simulink model "finalcode"  (R2020a)
settings: Solver=FixedStepDiscrete  StartTime=0.0  StopTime=1  FixedStep=0.0005  RelTol=1e-3  EnableMultiTasking=on
undefined symbols (not defined in the file): acc_calmax1, acc_calmax2, acc_calmin1, acc_calmin2, akemancanshu, angle_middle, bre, bre_calmax, bre_calmin, chasuniujvvvv_hou, chasuniujvvvv_qian, chasuuuu, ecucoder_acal, I_AN01_5K1, I_AN03_5V, I_AN04_5V, kd, kddd, ki, kiii, kp, kppp, leftmax, O_SW06_HS1A, P11111, P22222, PIDmodel, PPPP, rightmax, slip, slip_big, slip_little, slipmodel, T_add, T_del, tiaoshi, TTTTTyouren, vvvv, zhiling
libraries: ec5744lib x305, canmsglib x97, simulink x23
(part 7 of 11)

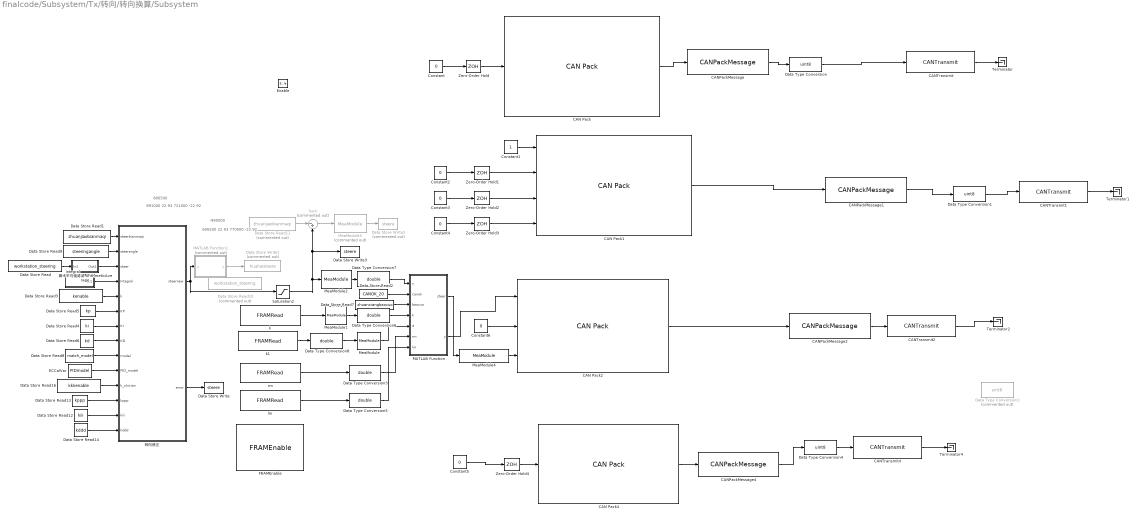
== system finalcode/Subsystem/Tx/转向/转向换算/Subsystem ==
  note: 606500  22.93
      | 770000  -22.92
  note: -990000
  note: 891000  22.93
      | 721000  -22.92
  note: 806500
  Enable : EnablePort
  CAN Pack : canmsglib/CAN Pack  CANdbFile=C:\Users\Liu keliang\Desktop\HRT2023\HRT23赛季刘科良\CANdbc\steering.dbc  MsgList=(none)  MsgName=enable123  MsgIDType=Standard (11-bit identifier)  MsgIdentifier=291  MsgLength=1  Remote=off  ApplyMinMax=off  BusOutput=off  SignalInfo={'enable123','0','8','LE','unsigned','Standard','0','1','0','0','255'}
      settings: SourceProductBaseCode=ME,XP,VN  DataFormat=CANdb specified signals
  CAN Pack1 : canmsglib/CAN Pack  CANdbFile=C:\Users\Liu keliang\Desktop\HRT2023\HRT23赛季刘科良\CANdbc\steering.dbc  MsgList=(none)  MsgName=enable0  MsgIDType=Standard (11-bit identifier)  MsgIdentifier=0  MsgLength=8  Remote=off  ApplyMinMax=off  BusOutput=off  SignalInfo={'enable_00','0','16','LE','unsigned','Standard','0','1','0','0','65535';'enable_00_Copy_1','16','16','LE','unsigned','Standard','0','1','0','0','65535';'enable_00_Copy_2','32','16','LE','unsigned','Standard','0','1','0','0','65535';'enable_00_Copy_3','48','16','LE','unsigned','Standard','0','1','0','0','65535'}
      settings: SourceProductBaseCode=ME,XP,VN  DataFormat=CANdb specified signals
  CAN Pack2 : canmsglib/CAN Pack  CANdbFile=C:\Users\Liu keliang\Desktop\HRT2023\HRT23赛季刘科良\CANdbc\steering.dbc  MsgList=(none)  MsgName=enable401  MsgIDType=Standard (11-bit identifier)  MsgIdentifier=1025  MsgLength=6  Remote=off  ApplyMinMax=off  BusOutput=off  SignalInfo={'enable401','0','8','LE','unsigned','Standard','0','1','0','0','255';'enable401_Copy_1','8','8','LE','unsigned','Standard','0','1','0','0','255';'enable401_Copy_2','16','32','LE','signed','Standard','0','1','0','-2147483648','2147483647'}
      settings: SourceProductBaseCode=ME,XP,VN  DataFormat=CANdb specified signals
  CAN Pack4 : canmsglib/CAN Pack  CANdbFile=C:\Users\Liu keliang\Desktop\HRT2023\HRT23赛季刘科良\CANdbc\steering.dbc  MsgList=(none)  MsgName=enable80  MsgIDType=Standard (11-bit identifier)  MsgIdentifier=128  MsgLength=1  Remote=off  ApplyMinMax=off  BusOutput=off  SignalInfo={'dingshi','0','8','LE','unsigned','Standard','0','1','0','0','255'}
      settings: SourceProductBaseCode=ME,XP,VN  DataFormat=CANdb specified signals
  CANPackMessage : ec5744lib/RapidECU_U4B/04CANCommunication/CANPackMessage  datalength=1  sampletime=-1
      settings: SourceProductName=ECUCoder for MPC5744
  CANPackMessage1 : ec5744lib/RapidECU_U4B/04CANCommunication/CANPackMessage  datalength=8  sampletime=-1
      settings: SourceProductName=ECUCoder for MPC5744
  CANPackMessage2 : ec5744lib/RapidECU_U4B/04CANCommunication/CANPackMessage  datalength=6  sampletime=-1
      settings: SourceProductName=ECUCoder for MPC5744
  CANPackMessage4 : ec5744lib/RapidECU_U4B/04CANCommunication/CANPackMessage  datalength=1  sampletime=-1
      settings: SourceProductName=ECUCoder for MPC5744
  CANTransmit : ec5744lib/RapidECU_U4B/04CANCommunication/CANTransmit  canmodule=2  canbuffer=15  canmessageid=hex2dec('123')  canmessagetype=Standard(11-bit ID)  datalength=1  sampletime=-1
      settings: SourceProductName=ECUCoder for MPC5744
  CANTransmit1 : ec5744lib/RapidECU_U4B/04CANCommunication/CANTransmit  canmodule=2  canbuffer=56  canmessageid=hex2dec('00')  canmessagetype=Standard(11-bit ID)  datalength=8  sampletime=-1
      settings: SourceProductName=ECUCoder for MPC5744
  CANTransmit2 : ec5744lib/RapidECU_U4B/04CANCommunication/CANTransmit  canmodule=2  canbuffer=57  canmessageid=hex2dec('401')  canmessagetype=Standard(11-bit ID)  datalength=6  sampletime=-1
      settings: SourceProductName=ECUCoder for MPC5744
  CANTransmit4 : ec5744lib/RapidECU_U4B/04CANCommunication/CANTransmit  canmodule=2  canbuffer=58  canmessageid=hex2dec('80')  canmessagetype=Standard(11-bit ID)  datalength=1  sampletime=-1
      settings: SourceProductName=ECUCoder for MPC5744
  Constant : Constant  Value=0  SampleTime=-1
  Constant1 : Constant  SampleTime=-1
  Constant{2..4,6} (4 alike) : Constant  Value=0
  Constant5 : Constant  Value=0  SampleTime=-1
  Data Store Read : DataStoreRead  DataStoreName=workstation_steering
  Data Store Read1 : DataStoreRead  DataStoreName=zhuanjiaobianmaqi
  Data Store Read10 : DataStoreRead  Commented=on  DataStoreName=workstation_steering
  Data Store Read11 : DataStoreRead  Commented=on  DataStoreName=zhuanjiaobianmaqi
  Data Store Read12 : DataStoreRead  DataStoreName=kiii
  Data Store Read13 : DataStoreRead  DataStoreName=kppp
  Data Store Read14 : DataStoreRead  DataStoreName=kddd
  Data Store Read16 : DataStoreRead  DataStoreName=kkkenable
  Data Store Read2 : DataStoreRead  DataStoreName=CANOK_20
  Data Store Read3 : DataStoreRead  DataStoreName=kenable
  Data Store Read4 : DataStoreRead  DataStoreName=ki
  Data Store Read5 : DataStoreRead  DataStoreName=kp
  Data Store Read6 : DataStoreRead  DataStoreName=kd
  Data Store Read7 : DataStoreRead  DataStoreName=zhuanxiangbaocuo
  Data Store Read8 : DataStoreRead  DataStoreName=match_model
  Data Store Read9 : DataStoreRead  DataStoreName=steeringangle
  Data Store Write : DataStoreWrite  DataStoreName=steere
  Data Store Write1 : DataStoreWrite  Commented=on  DataStoreName=huahaisteere
  Data Store Write2 : DataStoreWrite  Commented=on  DataStoreName=steere
  Data Store Write3 : DataStoreWrite  DataStoreName=steere
  Data Type Conversion : DataTypeConversion  OutDataTypeStr=uint8
  Data Type Conversion1 : DataTypeConversion  OutDataTypeStr=uint8
  Data Type Conversion2 : DataTypeConversion  Commented=on  OutDataTypeStr=uint8
  Data Type Conversion{3,5..8} (5 alike) : DataTypeConversion  OutDataTypeStr=double
  Data Type Conversion4 : DataTypeConversion  OutDataTypeStr=uint8
  ECCalVar : Constant  InitFcn=ecucoder_acal;  Value=PIDmodel  OutDataTypeStr=Inherit: Inherit via back propagation  SampleTime=-1
  FRAMEnable : ec5744lib/RapidECU_U4B/12EEModule/FRAMEnable  framenable=on
      settings: SourceProductName=ECUCoder for MPC5744
  MATLAB Function : MATLAB Function  TreatAsAtomicUnit=on
  MATLAB Function1 : MATLAB Function  Commented=on  TreatAsAtomicUnit=on
  MeaModule : ec5744lib/RapidECU_U4B/07Calibration/MeaModule  signal=d
      settings: SourceProductName=ECUCoder for MPC5744
  MeaModule1 : ec5744lib/RapidECU_U4B/07Calibration/MeaModule  signal=k
      settings: SourceProductName=ECUCoder for MPC5744
  MeaModule2 : ec5744lib/RapidECU_U4B/07Calibration/MeaModule  signal=steer_toworkstation
      settings: SourceProductName=ECUCoder for MPC5744
  MeaModule3 : ec5744lib/RapidECU_U4B/07Calibration/MeaModule  Commented=on  signal=steer_error
      settings: SourceProductName=ECUCoder for MPC5744
  MeaModule4 : ec5744lib/RapidECU_U4B/07Calibration/MeaModule  signal=zhuanjiaoshuzhi
      settings: SourceProductName=ECUCoder for MPC5744
  Saturation2 : Saturate  UpperLimit=25  LowerLimit=-25
  Sum : Sum  Commented=on  Inputs=|-+
  Terminator{,1..2,4} (4 alike) : Terminator
  Zero-Order Hold{,1..4} (5 alike) : ZeroOrderHold  SampleTime=-1
  integral : Subsystem
  k : ec5744lib/RapidECU_U4B/12EEModule/FRAMRead  buffer=0  sampletime=-1
      settings: SourceProductName=ECUCoder for MPC5744
  k1 : ec5744lib/RapidECU_U4B/12EEModule/FRAMRead  buffer=9  sampletime=-1
      settings: SourceProductName=ECUCoder for MPC5744
  lm : ec5744lib/RapidECU_U4B/12EEModule/FRAMRead  buffer=11  sampletime=-1
      settings: SourceProductName=ECUCoder for MPC5744
  rm : ec5744lib/RapidECU_U4B/12EEModule/FRAMRead  buffer=10  sampletime=-1
      settings: SourceProductName=ECUCoder for MPC5744
  算术平均值滤波 ArithmeticAverage : Subsystem
  转向修正 : MATLAB Function  TreatAsAtomicUnit=on
  wires:
  CANTransmit/1 -> Terminator/1
  Zero-Order Hold2/1 -> CAN Pack1/3
  MATLAB Function/2(y) -> CAN Pack2/1
  CAN Pack1/1 -> CANPackMessage1/1
  CANTransmit2/1 -> Terminator2/1
  CANPackMessage4/1 -> Data Type Conversion4/1
  CAN Pack2/1 -> CANPackMessage2/1
  CANTransmit1/1 -> Terminator1/1
  Constant/1 -> Zero-Order Hold/1
  Data Type Conversion1/1 -> CANTransmit1/1
  Constant6/1 -> CAN Pack2/2
  CANTransmit4/1 -> Terminator4/1
  Data Type Conversion/1 -> CANTransmit/1
  Zero-Order Hold/1 -> CAN Pack/1
  CANPackMessage/1 -> Data Type Conversion/1
  Data Type Conversion4/1 -> CANTransmit4/1
  Constant4/1 -> Zero-Order Hold3/1
  CAN Pack/1 -> CANPackMessage/1
  CANPackMessage1/1 -> Data Type Conversion1/1
  Constant5/1 -> Zero-Order Hold4/1
  CAN Pack4/1 -> CANPackMessage4/1
  Constant3/1 -> Zero-Order Hold2/1
  Constant2/1 -> Zero-Order Hold1/1
  Constant1/1 -> CAN Pack1/1
  Zero-Order Hold4/1 -> CAN Pack4/1
  Zero-Order Hold1/1 -> CAN Pack1/2
  CANPackMessage2/1 -> CANTransmit2/1
  Zero-Order Hold3/1 -> CAN Pack1/4
  MATLAB Function/1(steer) -> MeaModule4/1
  Data Store Read/1 -> 算术平均值滤波 ArithmeticAverage/1(In1)
  Data Store Read1/1 -> 转向修正/1(steerbianmaqi)
  转向修正/2(error) -> Data Store Write/1
  Data Store Read2/1 -> MATLAB Function/2(canok)
  Data Store Read5/1 -> 转向修正/6(KP)
  Data Store Read4/1 -> 转向修正/7(KI)
  Data Store Read3/1 -> 转向修正/5(k)
  Data Store Read6/1 -> 转向修正/8(KD)
  MATLAB Function1/1(y) -> Data Store Write1/1
  Data Store Read7/1 -> MATLAB Function/3(baocuo)
  Data Store Read8/1 -> 转向修正/9(model)
  Data Store Read9/1 -> 转向修正/2(steerangle)
  rm/1 -> Data Type Conversion3/1
  lm/1 -> Data Type Conversion5/1
  MeaModule/1 -> MATLAB Function/5(d)
  k/1 -> MeaModule1/1
  MeaModule1/1 -> Data Type Conversion6/1
  转向修正/1(steernew) -> MATLAB Function1/1(u), Saturation2/1
  MeaModule2/1 -> Data Type Conversion7/1
  Data Store Read11/1 -> Sum/1
  Sum/1 -> MeaModule3/1
  MeaModule3/1 -> Data Store Write2/1
  Data Type Conversion3/1 -> MATLAB Function/6(rm)
  Data Type Conversion5/1 -> MATLAB Function/7(lm)
  Data Type Conversion6/1 -> MATLAB Function/4(k)
  MeaModule4/1 -> CAN Pack2/3
  Data Type Conversion7/1 -> MATLAB Function/1(x)
  ECCalVar/1 -> 转向修正/10(PID_model)
  integral/1(Out1) -> 转向修正/4(Integral)
  算术平均值滤波 ArithmeticAverage/1(Out1) -> 转向修正/3(steer)
  k1/1 -> Data Type Conversion8/1
  Data Type Conversion8/1 -> MeaModule/1
  Data Store Read16/1 -> 转向修正/11(k_zhixian)
  Data Store Read13/1 -> 转向修正/12(kppp)
  Data Store Read12/1 -> 转向修正/13(kiii)
  Data Store Read14/1 -> 转向修正/14(kddd)
  Saturation2/1 -> Sum/2, Data Store Write3/1, MeaModule2/1

== system finalcode/Subsystem/Tx/转向/转向换算/Subsystem1 ==
  y1 : Inport
  y2 : Inport  Port=2
  Enable : EnablePort
  CAN Pack5 : canmsglib/CAN Pack  CANdbFile=C:\Users\Liu keliang\Desktop\HRT2023\HRT23赛季刘科良\CANdbc\zhuanxiangresetting.dbc  MsgList=(none)  MsgName=reseting  MsgIDType=Standard (11-bit identifier)  MsgIdentifier=1537  MsgLength=8  Remote=off  ApplyMinMax=off  BusOutput=off  SignalInfo={'reseting1','0','32','LE','unsigned','Standard','0','1','0','-Inf','Inf';'reseting2','32','32','LE','unsigned','Standard','0','1','0','-Inf','Inf'}
      settings: SourceProductBaseCode=ME,XP,VN  DataFormat=CANdb specified signals
  CANPackMessage3 : ec5744lib/RapidECU_U4B/04CANCommunication/CANPackMessage  datalength=8  sampletime=-1
      settings: SourceProductName=ECUCoder for MPC5744
  CANTransmit3 : ec5744lib/RapidECU_U4B/04CANCommunication/CANTransmit  canmodule=2  canbuffer=60  canmessageid=hex2dec('601')  canmessagetype=Standard(11-bit ID)  datalength=8  sampletime=-1
      settings: SourceProductName=ECUCoder for MPC5744
  Data Type Conversion3 : DataTypeConversion  OutDataTypeStr=uint8
  Terminator3 : Terminator
  wires:
  CAN Pack5/1 -> CANPackMessage3/1
  y1/1 -> CAN Pack5/1
  CANTransmit3/1 -> Terminator3/1
  Data Type Conversion3/1 -> CANTransmit3/1
  CANPackMessage3/1 -> Data Type Conversion3/1
  y2/1 -> CAN Pack5/2

== system finalcode/Subsystem/run/analog_input/无人意图转译/无人 ==
  Data Store Write : DataStoreWrite  DataStoreName=escmax
  Max : MinMax  Function=max  Inputs=4
  Subsystem1 : Subsystem
  右前油压 : DataStoreWrite  DataStoreName=oral_pressure_rightfront
  右后油压 : DataStoreWrite  DataStoreName=oral_pressure_rightbehind
  左前油压 : DataStoreWrite  DataStoreName=oral_pressure_leftfront
  左后油压 : DataStoreWrite  DataStoreName=oral_pressure_leftbehind
  期望加速度 : DataStoreWrite  Commented=on  DataStoreName=acc_expired
  期望纵向加速度 : Outport
  wires:
  Subsystem1/1(期望纵向加速度) -> 期望纵向加速度/1, 期望加速度/1
  Subsystem1/2(输出左前制动力) -> Max/1, 左前油压/1
  Subsystem1/4(输出左后制动力) -> Max/3, 左后油压/1
  Subsystem1/3(输出右前制动力) -> Max/2, 右前油压/1
  Subsystem1/5(输出右后制动力) -> Max/4, 右后油压/1
  Max/1 -> Data Store Write/1

== system finalcode/Subsystem/run/analog_input/有人/Subsystem1 ==
  note: 标定
  acc_signal : Inport
  Constant : Constant  Value=0
  Data Store Read : DataStoreRead  DataStoreName=V_Kalman
  Data Type Conversion : DataTypeConversion  OutMin=[0]  OutMax=[1]  OutDataTypeStr=double
  Divide1 : Product  Inputs=**  OutDataTypeStr=uint16
  ECCalVar : Constant  InitFcn=ecucoder_acal;  Value=T_add  OutDataTypeStr=Inherit: Inherit via back propagation  SampleTime=-1
  ECCalVar1 : Constant  InitFcn=ecucoder_acal;  Value=T_del  OutDataTypeStr=Inherit: Inherit via back propagation  SampleTime=-1
  ECCalVar2 : Constant  InitFcn=ecucoder_acal;  Value=zhiling  OutDataTypeStr=Inherit: Inherit via back propagation  SampleTime=-1
  MATLAB Function : MATLAB Function  TreatAsAtomicUnit=on
  MATLAB Function1 : MATLAB Function  TreatAsAtomicUnit=on
  Saturation3 : Saturate  UpperLimit=2100  LowerLimit=0
  Saturation4 : Saturate  UpperLimit=1  LowerLimit=0
  Sum : Sum  Inputs=|++-
  Sum1 : Sum  Inputs=+--
  normal : MATLAB Function  Commented=on  TreatAsAtomicUnit=on
  TP : Outport
  wires:
  Data Type Conversion/1 -> Saturation4/1
  acc_signal/1 -> Data Type Conversion/1
  Saturation4/1 -> Divide1/2
  Sum/1 -> Divide1/1
  ECCalVar1/1 -> Sum/3
  ECCalVar/1 -> Sum/1
  Saturation3/1 -> Sum/2
  Data Store Read/1 -> MATLAB Function/1(v)
  MATLAB Function/1(T) -> Saturation3/1
  Divide1/1 -> Sum1/1
  Constant/1 -> Sum1/2
  Sum1/1 -> MATLAB Function1/1(T)
  MATLAB Function1/1(TP) -> TP/1
  ECCalVar2/1 -> Sum1/3

== system finalcode/Subsystem/run/analog_input/有人/功率限制 ==
  M_zuoqian : Inport
  M_youqian : Inport  Port=2
  M_zuohou : Inport  Port=3
  M_youhou : Inport  Port=4
  Data Store Read4 : DataStoreRead  DataStoreName=dianji_velcoity_zuoqian
  Data Store Read5 : DataStoreRead  DataStoreName=dianji_velcoity_youhou
  Data Store Read6 : DataStoreRead  DataStoreName=dianji_velcoity_youqian
  Data Store Read7 : DataStoreRead  DataStoreName=dianji_velcoity_zuohou
  Data Store Write : DataStoreWrite  DataStoreName=Tzuoqian
  Data Store Write1 : DataStoreWrite  DataStoreName=Tyouqian
  Data Store Write2 : DataStoreWrite  DataStoreName=Tzuohou
  Data Store Write3 : DataStoreWrite  DataStoreName=Tyouhou
  MATLAB Function : MATLAB Function  TreatAsAtomicUnit=on
  Product{,1..7} (8 alike) : Product
  wires:
  M_youqian/1 -> Product5/1, Product1/1
  M_zuohou/1 -> Product6/1, Product2/1
  M_youhou/1 -> Product7/1, Product3/1
  Data Store Read4/1 -> Product/2
  Data Store Read7/1 -> Product2/2
  Data Store Read5/1 -> Product3/2
  Data Store Read6/1 -> Product1/2
  Product/1 -> MATLAB Function/1(u1)
  Product1/1 -> MATLAB Function/2(u2)
  Product2/1 -> MATLAB Function/3(u3)
  Product3/1 -> MATLAB Function/4(u4)
  MATLAB Function/1(y) -> Product7/2, Product6/2, Product5/2, Product4/2
  M_zuoqian/1 -> Product4/1, Product/1
  Product4/1 -> Data Store Write/1
  Product5/1 -> Data Store Write1/1
  Product6/1 -> Data Store Write2/1
  Product7/1 -> Data Store Write3/1

== system finalcode/Subsystem/run/analog_input/有人/功率限制jiandan ==
  M_zuoqian : Inport
  M_youqian : Inport  Port=2
  M_zuohou : Inport  Port=3
  M_youhou : Inport  Port=4
  Data Store Read4 : DataStoreRead  DataStoreName=dianji_velcoity_zuoqian
  Data Store Read5 : DataStoreRead  DataStoreName=dianji_velcoity_youhou
  Data Store Read6 : DataStoreRead  DataStoreName=dianji_velcoity_youqian
  Data Store Read7 : DataStoreRead  DataStoreName=dianji_velcoity_zuohou
  Data Store Write : DataStoreWrite  DataStoreName=Tzuoqian
  Data Store Write1 : DataStoreWrite  DataStoreName=Tyouqian
  Data Store Write2 : DataStoreWrite  DataStoreName=Tzuohou
  Data Store Write3 : DataStoreWrite  DataStoreName=Tyouhou
  MATLAB Function : MATLAB Function  TreatAsAtomicUnit=on
  Product{,1..7} (8 alike) : Product
  Saturation{1..4} (4 alike) : Saturate  UpperLimit=2100  LowerLimit=0
  wires:
  M_youqian/1 -> Product5/1, Product1/1
  M_zuohou/1 -> Product6/1, Product2/1
  M_youhou/1 -> Product7/1, Product3/1
  Data Store Read4/1 -> Product/2
  Data Store Read7/1 -> Product2/2
  Data Store Read5/1 -> Product3/2
  Data Store Read6/1 -> Product1/2
  Product/1 -> MATLAB Function/1(u1)
  Product1/1 -> MATLAB Function/2(u2)
  Product2/1 -> MATLAB Function/3(u3)
  Product3/1 -> MATLAB Function/4(u4)
  MATLAB Function/1(y) -> Product7/2, Product6/2, Product5/2, Product4/2
  M_zuoqian/1 -> Product4/1, Product/1
  Product4/1 -> Saturation3/1
  Saturation3/1 -> Data Store Write/1
  Product5/1 -> Saturation1/1
  Saturation1/1 -> Data Store Write1/1
  Product6/1 -> Saturation2/1
  Saturation2/1 -> Data Store Write2/1
  Product7/1 -> Saturation4/1
  Saturation4/1 -> Data Store Write3/1

== system finalcode/Subsystem/run/analog_input/有人/扭矩分配 ==
  note: 前后扭矩分配k
  fengzhiniuju : Inport
  Constant2 : Constant  Value=10
  Data Store Read7 : DataStoreRead  DataStoreName=acc_calibration
  Enabled Subsystem : Subsystem  TreatAsAtomicUnit=on
  MATLAB Function : MATLAB Function  TreatAsAtomicUnit=on
  MATLAB Function3 : MATLAB Function  TreatAsAtomicUnit=on
  Saturation : Saturate  UpperLimit=2100  LowerLimit=0
  Saturation1 : Saturate  UpperLimit=2100  LowerLimit=0
  zuoqian : Outport
  youqian : Outport  Port=2
  zuohou : Outport  Port=3
  youhou : Outport  Port=4
  wires:
  MATLAB Function/1(M_qian) -> Saturation1/1
  fengzhiniuju/1 -> MATLAB Function/1(M)
  MATLAB Function/2(M_hou) -> Saturation/1
  Constant2/1 -> MATLAB Function/3(k)
  MATLAB Function3/1(youhou) -> youhou/1
  MATLAB Function3/2(youqian) -> youqian/1
  MATLAB Function3/3(zuohou) -> zuohou/1
  MATLAB Function3/4(zuoqian) -> zuoqian/1
  Data Store Read7/1 -> MATLAB Function/2(ax)
  Enabled Subsystem/1(y) -> MATLAB Function3/3(M)
  Saturation1/1 -> MATLAB Function3/1(M_qian)
  Saturation/1 -> MATLAB Function3/2(M_hou)

== system finalcode/Subsystem/run/analog_input/有人/扭矩分配jiandan ==
  note: 后面加入载荷转移，向心差扭
  note: 前后扭矩分配k
  fengzhiniuju : Inport
  Constant2 : Constant
  Constant3 : Constant
  Data Store Read2 : DataStoreRead  Commented=on  DataStoreName=shucai_ax
  Data Store Read3 : DataStoreRead  Commented=on  DataStoreName=shucai_ay
  MATLAB Function1 : MATLAB Function  Commented=on  TreatAsAtomicUnit=on
  MATLAB Function3 : MATLAB Function  TreatAsAtomicUnit=on
  M_back : Constant  Value=1.3
  M_front : Constant  Value=0.7
  Product1 : Product
  Product2 : Product
  k : Constant  Value=0
  zuoqian : Outport
  youqian : Outport  Port=2
  zuohou : Outport  Port=3
  youhou : Outport  Port=4
  wires:
  MATLAB Function3/1(youhou) -> youhou/1
  MATLAB Function3/2(youqian) -> youqian/1
  MATLAB Function3/3(zuohou) -> zuohou/1
  MATLAB Function3/4(zuoqian) -> zuoqian/1
  k/1 -> MATLAB Function3/3(M)
  Product1/1 -> MATLAB Function3/1(M_qian)
  Product2/1 -> MATLAB Function3/2(M_hou)
  M_front/1 -> Product1/2
  Constant2/1 -> MATLAB Function3/5(zuo)
  Constant3/1 -> MATLAB Function3/4(you)
  fengzhiniuju/1 -> Product2/2, MATLAB Function1/1(fengzhiniuju), Product1/1
  M_back/1 -> Product2/1
  Data Store Read2/1 -> MATLAB Function1/2(ax)
  Data Store Read3/1 -> MATLAB Function1/3(ay)

== system finalcode/Subsystem/run/analog_input/有人/踏板标定 ==
  AnalogInput : ec5744lib/RapidECU_U4B/01BasicInput/AnalogInput  channel=52:I_AN03_5V  sampletime=-1
      settings: SourceProductName=ECUCoder for MPC5744
  AnalogInput1 : ec5744lib/RapidECU_U4B/01BasicInput/AnalogInput  channel=53:I_AN04_5V  sampletime=-1
      settings: SourceProductName=ECUCoder for MPC5744
  AnalogInput2 : ec5744lib/RapidECU_U4B/01BasicInput/AnalogInput  Commented=on  channel=34:I_AN01_5K1  sampletime=-1
      settings: SourceProductName=ECUCoder for MPC5744
  Data Store Write1 : DataStoreWrite  DataStoreName=acc_calibration
  Data Store Write2 : DataStoreWrite  DataStoreName=bre_calibration
  ECCalVar1 : Constant  InitFcn=ecucoder_acal;  Value=acc_calmax1  OutDataTypeStr=double  SampleTime=-1
  ECCalVar2 : Constant  InitFcn=ecucoder_acal;  Value=acc_calmin1  OutDataTypeStr=double  SampleTime=-1
  ECCalVar3 : Constant  InitFcn=ecucoder_acal;  Value=acc_calmax2  OutDataTypeStr=double  SampleTime=-1
  ECCalVar4 : Constant  InitFcn=ecucoder_acal;  Value=acc_calmin2  OutDataTypeStr=double  SampleTime=-1
  ECCalVar5 : Constant  Commented=on  InitFcn=ecucoder_acal;  Value=bre_calmax  OutDataTypeStr=double  SampleTime=-1
  ECCalVar6 : Constant  Commented=on  InitFcn=ecucoder_acal;  Value=bre_calmin  OutDataTypeStr=double  SampleTime=-1
  ECCalVar7 : Constant  InitFcn=ecucoder_acal;  Value=bre  OutDataTypeStr=double  SampleTime=-1
  FRAMEnable : ec5744lib/RapidECU_U4B/12EEModule/FRAMEnable  Commented=on  framenable=off
      settings: SourceProductName=ECUCoder for MPC5744
  MATLAB Function : MATLAB Function  TreatAsAtomicUnit=on
  MATLAB Function1 : MATLAB Function  Commented=on  TreatAsAtomicUnit=on
  MATLAB Function2 : MATLAB Function  TreatAsAtomicUnit=on
  MeaModule1 : ec5744lib/RapidECU_U4B/07Calibration/MeaModule  signal=acc_ori_line1
      settings: SourceProductName=ECUCoder for MPC5744
  MeaModule2 : ec5744lib/RapidECU_U4B/07Calibration/MeaModule  signal=acc_ori_line2
      settings: SourceProductName=ECUCoder for MPC5744
  MeaModule3 : ec5744lib/RapidECU_U4B/07Calibration/MeaModule  signal=guiyi
      settings: SourceProductName=ECUCoder for MPC5744
  MeaModule5 : ec5744lib/RapidECU_U4B/07Calibration/MeaModule  Commented=on  signal=bre_ori_sig
      settings: SourceProductName=ECUCoder for MPC5744
  MeaModule6 : ec5744lib/RapidECU_U4B/07Calibration/MeaModule  signal=acc_result2
      settings: SourceProductName=ECUCoder for MPC5744
  MeaModule8 : ec5744lib/RapidECU_U4B/07Calibration/MeaModule  signal=acc_result1
      settings: SourceProductName=ECUCoder for MPC5744
  MeaModule9 : ec5744lib/RapidECU_U4B/07Calibration/MeaModule  signal=bre_result
      settings: SourceProductName=ECUCoder for MPC5744
  Saturation4 : Saturate  UpperLimit=1  LowerLimit=0
  Subsystem : Subsystem  Commented=on
  Subsystem1 : Subsystem  Commented=on
  无人制动标志位 : DataStoreRead  DataStoreName=wurenzhidongdeng
  算术平均值滤波 ArithmeticAverage1 : Subsystem
  踏板冲突 : MATLAB Function  TreatAsAtomicUnit=on
  踏板冲突1 : MATLAB Function  Commented=on  TreatAsAtomicUnit=on
  acc : Outport
  bre : Outport  Port=2
  wires:
  AnalogInput/1 -> MeaModule1/1
  AnalogInput2/1 -> MeaModule5/1
  MeaModule5/1 -> MATLAB Function1/1(u)
  AnalogInput1/1 -> MeaModule2/1
  MeaModule1/1 -> MATLAB Function/1(u)
  MeaModule2/1 -> MATLAB Function2/1(u)
  MeaModule9/1 -> bre/1, Data Store Write2/1, 踏板冲突/3(bre_ori_sig)
  ECCalVar3/1 -> MATLAB Function2/3(max)
  MATLAB Function2/1(y) -> MeaModule6/1
  ECCalVar1/1 -> MATLAB Function/3(max)
  ECCalVar4/1 -> MATLAB Function2/2(min)
  MATLAB Function/1(y) -> MeaModule8/1
  ECCalVar2/1 -> MATLAB Function/2(min)
  Subsystem1/1(y) -> Subsystem/Enable
  MeaModule6/1 -> 踏板冲突/2(acc_fin_sig2)
  ECCalVar6/1 -> MATLAB Function1/2(min)
  ECCalVar5/1 -> MATLAB Function1/3(max)
  踏板冲突/1(y) -> Saturation4/1
  MeaModule3/1 -> acc/1
  ECCalVar7/1 -> 踏板冲突/4(bre)
  无人制动标志位/1 -> MeaModule9/1
  Saturation4/1 -> Data Store Write1/1, 算术平均值滤波 ArithmeticAverage1/1(In1)
  MeaModule8/1 -> 踏板冲突/1(acc_fin_sig1)
  算术平均值滤波 ArithmeticAverage1/1(angle) -> MeaModule3/1

== system finalcode/Subsystem/run/analog_input/有人/限滑 ==
  note: 左转是正
  zuoqian : Inport
  youqian : Inport  Port=2
  zuohou : Inport  Port=3
  youhou : Inport  Port=4
  Data Store Read : DataStoreRead  DataStoreName=shucai_ax
  Enabled Subsystem : Subsystem  TreatAsAtomicUnit=on
  Enabled Subsystem1 : Subsystem  TreatAsAtomicUnit=on
  MATLAB Function : MATLAB Function  TreatAsAtomicUnit=on
  Switch{,1..3} (4 alike) : Switch  Criteria=u2 > Threshold  Threshold=0.5
  M_zuoqian : Outport
  M_youqian : Outport  Port=2
  M_zuohou : Outport  Port=3
  M_youhou : Outport  Port=4
  wires:
  zuoqian/1 -> Enabled Subsystem1/1(zuoqian), Enabled Subsystem/1(zuoqian)
  zuohou/1 -> Enabled Subsystem1/3(zuohou), Enabled Subsystem/3(zuohou)
  youhou/1 -> Enabled Subsystem1/4(youhou), Enabled Subsystem/4(youhou)
  youqian/1 -> Enabled Subsystem1/2(youqian), Enabled Subsystem/2(youqian)
  Data Store Read/1 -> MATLAB Function/1(u)
  MATLAB Function/1(y) -> Switch2/2, Switch3/2, Switch1/2, Switch/2
  Enabled Subsystem/1(M_zuoqian) -> Switch/1
  Enabled Subsystem1/1(M_zuoqian) -> Switch/3
  Enabled Subsystem/4(M_youhou) -> Switch3/1
  Enabled Subsystem1/4(M_youhou) -> Switch3/3
  Enabled Subsystem1/3(M_zuohou) -> Switch2/3
  Enabled Subsystem/3(M_zuohou) -> Switch2/1
  Enabled Subsystem/2(M_youqian) -> Switch1/1
  Enabled Subsystem1/2(M_youqian) -> Switch1/3
  Switch/1 -> M_zuoqian/1
  Switch3/1 -> M_youhou/1
  Switch1/1 -> M_youqian/1
  Switch2/1 -> M_zuohou/1

== system finalcode/Subsystem/run/ctrl/Subsystem1/control_strategy ==
  TP : Inport
  Data Store Read1 : DataStoreRead  DataStoreName=workstation_steering
  Data Store Read2 : DataStoreRead  DataStoreName=slipyouhou
  Data Store Read4 : DataStoreRead  DataStoreName=workstation_steering
  Data Store Read5 : DataStoreRead  DataStoreName=slipzuohou
  Data Store Read6 : DataStoreRead  DataStoreName=slipyuoqian
  Data Store Read7 : DataStoreRead  DataStoreName=slipzuoqian
  E,H : MATLAB Function  Commented=on  TreatAsAtomicUnit=on
  MATLAB Function : MATLAB Function  Commented=on  TreatAsAtomicUnit=on
  MATLAB Function1 : MATLAB Function  TreatAsAtomicUnit=on
  MATLAB Function2 : MATLAB Function  Commented=on  TreatAsAtomicUnit=on
  MATLAB Function3 : MATLAB Function  TreatAsAtomicUnit=on
  MPC : MATLAB Function  Commented=on  TreatAsAtomicUnit=on
  Subsystem : Subsystem  Commented=on
  Switch{,1..3} (4 alike) : Switch  Criteria=u2 > Threshold
  差速 : Subsystem
  滑模控制 : MATLAB Function  TreatAsAtomicUnit=on
  限滑 : Subsystem
  youhou : Outport
  youqian : Outport  Port=2
  zuohou : Outport  Port=3
  zuoqian : Outport  Port=4
  wires:
  TP/1 -> 差速/1(u), 限滑/1(In1)
  Data Store Read4/1 -> MATLAB Function1/1(angle)
  MATLAB Function1/1(y) -> Switch2/2, Switch3/2, Switch1/2, Switch/2
  限滑/1(youhou) -> Switch/3
  限滑/2(youqian) -> Switch1/3
  限滑/3(zuohou) -> Switch2/3
  限滑/4(zuoqian) -> Switch3/3
  MATLAB Function2/1(A) -> E,H/1(A)
  MATLAB Function2/2(B) -> E,H/2(B)
  MATLAB Function2/3(Q) -> E,H/3(Q)
  MATLAB Function2/4(R) -> E,H/4(R)
  MATLAB Function2/5(F) -> E,H/5(F)
  MATLAB Function2/6(N) -> E,H/6(N)
  差速/1(youhou) -> Switch/1
  差速/2(youqian) -> Switch1/1
  差速/3(zuohou) -> Switch2/1
  差速/4(zuoqian) -> Switch3/1
  Data Store Read1/1 -> MATLAB Function3/1(angle)
  MATLAB Function3/1(y) -> 差速/Enable
  Data Store Read7/1 -> 滑模控制/1(slip_ratio_fl)
  Switch/1 -> 滑模控制/8(driver_torque_cmd_rr)
  Data Store Read2/1 -> 滑模控制/4(slip_ratio_rr)
  Data Store Read6/1 -> 滑模控制/2(slip_ratio_fr)
  Switch3/1 -> 滑模控制/5(driver_torque_cmd_fl)
  Data Store Read5/1 -> 滑模控制/3(slip_ratio_rl)
  Switch1/1 -> 滑模控制/6(driver_torque_cmd_fr)
  Switch2/1 -> 滑模控制/7(driver_torque_cmd_rl)
  滑模控制/4(torque_cmd_rr) -> youhou/1
  滑模控制/2(torque_cmd_fr) -> youqian/1
  滑模控制/3(torque_cmd_rl) -> zuohou/1
  滑模控制/1(torque_cmd_fl) -> zuoqian/1

== system finalcode/Subsystem/Rx/工作站/Subsystem1/Subsystem1/Subsystem ==
  ID : Inport
  msg : Inport  Port=2
  CAN Unpack : canmsglib/CAN Unpack  CANdbFile=C:\Users\Liu keliang\Desktop\HRT2023\HRT23赛季刘科良\CANdbc\INSWORKSTATION.dbc  MsgList=(none)  MsgName=ins  MsgIDType=Standard (11-bit identifier)  MsgIdentifier=33  MsgLength=8  SignalInfo={'Vx','32','16','LE','unsigned','Standard','0','1','0','0','65535';'Vy','48','16','LE','unsigned','Standard','0','1','0','0','65535';'ax','0','8','LE','signed','Standard','0','1','0','-128','127';'ay','8','16','LE','signed','Standard','0','1','0','-32768','32767';'az','24','8','LE','signed','Standard','0','1','0','-128','127'}  IDPort=off  TimestampPort=off  ErrorPort=off  RemotePort=off  LengthPort=off  StatusPort=off  ApplyMinMax=off
      settings: SourceProductBaseCode=ME,XP,VN  DataFormat=CANdb specified signals
  CANUnPackMessage : ec5744lib/RapidECU_U4B/04CANCommunication/CANUnPackMessage  datalength=8  canmessagetype=Standard(11-bit ID)  sampletime=-1
      settings: SourceProductName=ECUCoder for MPC5744
  Data Store Write1 : DataStoreWrite  DataStoreName=ACC_X
  Data Store Write2 : DataStoreWrite  DataStoreName=ACC_Y
  Data Store Write3 : DataStoreWrite  DataStoreName=ACC_Z
  Data Store Write4 : DataStoreWrite  DataStoreName=V_Y
  Data Store Write5 : DataStoreWrite  DataStoreName=V_X
  wires:
  msg/1 -> CANUnPackMessage/2
  CANUnPackMessage/1 -> CAN Unpack/1
  ID/1 -> CANUnPackMessage/1
  CAN Unpack/2 -> Data Store Write4/1
  CAN Unpack/1 -> Data Store Write5/1
  CAN Unpack/3 -> Data Store Write1/1
  CAN Unpack/5 -> Data Store Write3/1
  CAN Unpack/4 -> Data Store Write2/1

== system finalcode/Subsystem/Rx/工作站/Subsystem3/Subsystem/Subsystem ==
  Data Store Read : DataStoreRead  DataStoreName=CANOK_20
  Delay : Delay  DelayLength=1
  Delay1 : Delay
  Delay10 : Delay  DelayLength=11
  Delay11 : Delay  DelayLength=12
  Delay12 : Delay  DelayLength=13
  Delay13 : Delay  DelayLength=14
  Delay14 : Delay  DelayLength=15
  Delay15 : Delay  DelayLength=16
  Delay16 : Delay  DelayLength=17
  Delay17 : Delay  DelayLength=25
  Delay18 : Delay  DelayLength=18
  Delay19 : Delay  DelayLength=19
  Delay2 : Delay  DelayLength=3
  Delay20 : Delay  DelayLength=20
  Delay21 : Delay  DelayLength=21
  Delay22 : Delay  DelayLength=22
  Delay23 : Delay  DelayLength=26
  Delay24 : Delay  DelayLength=24
  Delay25 : Delay  DelayLength=27
  Delay3 : Delay  DelayLength=4
  Delay4 : Delay  DelayLength=5
  Delay5 : Delay  DelayLength=6
  Delay6 : Delay  DelayLength=7
  Delay7 : Delay  DelayLength=8
  Delay8 : Delay  DelayLength=9
  Delay9 : Delay  DelayLength=10
  OR : Logic  Operator=OR  Inputs=27  IconShape=distinctive  AllPortsSameDT=off  OutDataTypeStr=boolean
  Out1 : Outport
  wires:
  Delay2/1 -> OR/2
  Delay/1 -> OR/4
  Data Store Read/1 -> Delay23/1, Delay25/1, Delay17/1, Delay24/1, Delay22/1, Delay21/1, Delay20/1, Delay19/1, Delay18/1, Delay16/1, Delay15/1, Delay14/1, Delay13/1, Delay12/1, Delay11/1, Delay10/1, Delay8/1, Delay6/1, Delay5/1, Delay7/1, Delay9/1, OR/5, Delay3/1, Delay2/1, Delay1/1, Delay/1, Delay4/1
  Delay5/1 -> OR/7
  Delay1/1 -> OR/3
  Delay9/1 -> OR/11
  Delay7/1 -> OR/9
  Delay3/1 -> OR/1
  Delay8/1 -> OR/8
  Delay6/1 -> OR/6
  Delay4/1 -> OR/10
  OR/1 -> Out1/1
  Delay10/1 -> OR/12
  Delay11/1 -> OR/13
  Delay12/1 -> OR/14
  Delay13/1 -> OR/15
  Delay14/1 -> OR/16
  Delay15/1 -> OR/17
  Delay16/1 -> OR/18
  Delay18/1 -> OR/19
  Delay19/1 -> OR/20
  Delay20/1 -> OR/21
  Delay21/1 -> OR/22
  Delay22/1 -> OR/23
  Delay24/1 -> OR/24
  Delay17/1 -> OR/25
  Delay23/1 -> OR/27
  Delay25/1 -> OR/26

== system finalcode/Subsystem/Tx/TX控制器/扭矩/TEST/Subsystem ==
  Enable : EnablePort
  CAN Pack1 : canmsglib/CAN Pack  CANdbFile=C:\Users\Liu keliang\Desktop\HRT2023\HRT23赛季刘科良\CANdbc\TEST.dbc  MsgList=(none)  MsgName=TEST  MsgIDType=Standard (11-bit identifier)  MsgIdentifier=153  MsgLength=5  Remote=off  ApplyMinMax=off  BusOutput=off  SignalInfo={'M','16','8','LE','signed','Standard','0','1','0','-Inf','Inf';'X2D','32','8','LE','signed','Standard','0','1','0','-Inf','Inf';'a','0','8','LE','signed','Standard','0','1','0','-Inf','Inf';'deltv','8','8','LE','signed','Standard','0','1','0','-Inf','Inf';'niuju','24','8','LE','signed','Standard','0','1','0','-Inf','Inf'}
      settings: SourceProductBaseCode=ME,XP,VN  DataFormat=CANdb specified signals
  CANPackMessage1 : ec5744lib/RapidECU_U4B/04CANCommunication/CANPackMessage  datalength=5  sampletime=-1
      settings: SourceProductName=ECUCoder for MPC5744
  CANTransmit : ec5744lib/RapidECU_U4B/04CANCommunication/CANTransmit  canmodule=0  canbuffer=63  canmessageid=hex2dec('99')  canmessagetype=Standard(11-bit ID)  datalength=5  sampletime=-1
      settings: SourceProductName=ECUCoder for MPC5744
  Data Store Read : DataStoreRead  DataStoreName=a
  Data Store Read1 : DataStoreRead  DataStoreName=ve
  Data Store Read2 : DataStoreRead  DataStoreName=M
  Data Store Read3 : DataStoreRead  DataStoreName=acc
  Data Store Read4 : DataStoreRead  DataStoreName=dianji_velcoity_zuoqian
  Data Type Conversion1 : DataTypeConversion  OutDataTypeStr=uint8
  Terminator : Terminator
  wires:
  Data Store Read4/1 -> CAN Pack1/1
  CANTransmit/1 -> Terminator/1
  Data Store Read3/1 -> CAN Pack1/3
  CANPackMessage1/1 -> Data Type Conversion1/1
  Data Store Read2/1 -> CAN Pack1/5
  Data Type Conversion1/1 -> CANTransmit/1
  Data Store Read1/1 -> CAN Pack1/4
  Data Store Read/1 -> CAN Pack1/2
  CAN Pack1/1 -> CANPackMessage1/1

== system finalcode/Subsystem/Tx/TX控制器/控制器发送/184左前1/算术平均值滤波 ArithmeticAverage5 ==
  In1 : Inport
  Constant : Constant  Value=10
  Divide : Product  Inputs=*/
  Sum of Elements : Sum  Inputs=+
  Tapped Delay : simulink/Discrete/Tapped Delay  vinit=0.0  samptime=-1  NumDelays=10  DelayOrder=Oldest  includeCurrent=off
  angle : Outport
  wires:
  Tapped Delay/1 -> Sum of Elements/1
  In1/1 -> Tapped Delay/1
  Divide/1 -> angle/1
  Sum of Elements/1 -> Divide/1
  Constant/1 -> Divide/2

== system finalcode/Subsystem/Tx/TX控制器/控制器发送/184左前1/能量回收功率限制 ==
  note: Tniujv
  note: U
  note: Iq
  Constant1 : Constant  Value=2
  Constant24 : Constant  Value=1000
  Data Store Read1 : DataStoreRead  DataStoreName=er_T_lf
  Data Store Read2 : DataStoreRead  DataStoreName=match_model
  Data Store Read23 : DataStoreRead  DataStoreName=match_model
  Data Store Read25 : DataStoreRead  DataStoreName=er_v_lf
  Data Store Read3 : DataStoreRead  DataStoreName=oral_pressure_leftfront
  Data Store Read4 : DataStoreRead  DataStoreName=Power_recovery
  Data Store Read5 : DataStoreRead  DataStoreName=Negativ_T
  Data Store Read6 : DataStoreRead  DataStoreName=Power_recovery_xunji
  Data Store Read7 : DataStoreRead  DataStoreName=Power_recovery_zhixian
  Data Store Read8 : DataStoreRead  DataStoreName=workstation_status
  Divide : Product  Inputs=*/
  Divide1 : Product  Inputs=***/
  Divide2 : Product  Inputs=**
  Gain : Gain  Gain=100
  Gain1 : Gain  Gain=1.5
  MATLAB Function : MATLAB Function  TreatAsAtomicUnit=on
  MATLAB Function1 : MATLAB Function  TreatAsAtomicUnit=on
  MeaModule : ec5744lib/RapidECU_U4B/07Calibration/MeaModule  signal=NT3
      settings: SourceProductName=ECUCoder for MPC5744
  P功率 : MATLAB Function  TreatAsAtomicUnit=on
  Saturation : Saturate  UpperLimit=0  LowerLimit=-1500
  Saturation1 : Saturate  UpperLimit=1500  LowerLimit=-1500
  Saturation2 : Saturate  UpperLimit=0  LowerLimit=-1500
  Sqrt : Sqrt  SaturateOnIntegerOverflow=on
  扭矩常量Kr  N/A : Constant  Value=0.26
  油压传感器 : DataStoreRead  DataStoreName=ebszhidongyouya
  电压常数Ke V/kU/min : Constant  Value=18.8
  T : Outport
  wires:
  Data Store Read25/1 -> Divide1/1
  电压常数Ke V/kU/min/1 -> Divide1/2
  Constant24/1 -> Divide1/4
  Sqrt/1 -> Divide1/3
  Constant1/1 -> Sqrt/1
  油压传感器/1 -> MATLAB Function/1(youya)
  Divide1/1 -> Divide/2
  Divide/1 -> Divide2/1, MATLAB Function1/3(L_Iq)
  扭矩常量Kr  N/A/1 -> Divide2/2
  MATLAB Function/1(T) -> Gain1/1
  Data Store Read1/1 -> MATLAB Function1/2(Iq)
  Divide2/1 -> Gain/1
  Gain/1 -> Saturation1/1
  MATLAB Function1/1(T) -> Saturation2/1
  Data Store Read2/1 -> MATLAB Function/2(model)
  Data Store Read8/1 -> MATLAB Function/3(status)
  Data Store Read3/1 -> MATLAB Function/4(wurenyouya)
  Data Store Read5/1 -> MATLAB Function/5(Negativ_T)
  Saturation/1 -> MeaModule/1
  Gain1/1 -> Saturation/1
  Saturation1/1 -> MATLAB Function1/4(L_er_T)
  Saturation2/1 -> T/1
  P功率/1(y) -> Divide/1
  Data Store Read23/1 -> P功率/4(model)
  Data Store Read4/1 -> P功率/1(P)
  Data Store Read6/1 -> P功率/2(P1)
  MeaModule/1 -> MATLAB Function1/1(er_T)
  Data Store Read7/1 -> P功率/3(P2)

== system finalcode/Subsystem/Tx/TX控制器/控制器发送/185右前1/算术平均值滤波 ArithmeticAverage5 ==
  In1 : Inport
  Constant : Constant  Value=10
  Divide : Product  Inputs=*/
  Sum of Elements : Sum  Inputs=+
  Tapped Delay : simulink/Discrete/Tapped Delay  vinit=0.0  samptime=-1  NumDelays=10  DelayOrder=Oldest  includeCurrent=off
  angle : Outport
  wires:
  Tapped Delay/1 -> Sum of Elements/1
  In1/1 -> Tapped Delay/1
  Divide/1 -> angle/1
  Sum of Elements/1 -> Divide/1
  Constant/1 -> Divide/2

== system finalcode/Subsystem/Tx/TX控制器/控制器发送/185右前1/能量回收功率限制 ==
  note: U
  note: Iq
  Constant1 : Constant  Value=2
  Constant24 : Constant  Value=1000
  Data Store Read1 : DataStoreRead  DataStoreName=er_T_rf
  Data Store Read2 : DataStoreRead  DataStoreName=match_model
  Data Store Read23 : DataStoreRead  DataStoreName=match_model
  Data Store Read25 : DataStoreRead  DataStoreName=er_v_rf
  Data Store Read3 : DataStoreRead  DataStoreName=oral_pressure_rightfront
  Data Store Read4 : DataStoreRead  DataStoreName=Power_recovery
  Data Store Read5 : DataStoreRead  DataStoreName=Negativ_T
  Data Store Read6 : DataStoreRead  DataStoreName=Power_recovery_xunji
  Data Store Read7 : DataStoreRead  DataStoreName=Power_recovery_zhixian
  Data Store Read8 : DataStoreRead  DataStoreName=workstation_status
  Divide : Product  Inputs=*/
  Divide1 : Product  Inputs=***/
  Divide2 : Product  Inputs=**
  Gain : Gain  Gain=100
  Gain1 : Gain  Gain=1.5
  MATLAB Function : MATLAB Function  TreatAsAtomicUnit=on
  MATLAB Function1 : MATLAB Function  TreatAsAtomicUnit=on
  MATLAB Function2 : MATLAB Function  TreatAsAtomicUnit=on
  Saturation : Saturate  UpperLimit=0  LowerLimit=-1500
  Saturation1 : Saturate  UpperLimit=1500  LowerLimit=-1500
  Saturation2 : Saturate  UpperLimit=0  LowerLimit=-1500
  Sqrt : Sqrt  SaturateOnIntegerOverflow=on
  扭矩常量Kr  N/A : Constant  Value=0.26
  油压传感器 : DataStoreRead  DataStoreName=ebszhidongyouya
  电压常数Ke V/kU/min : Constant  Value=18.8
  T : Outport
  wires:
  Data Store Read25/1 -> Divide1/1
  电压常数Ke V/kU/min/1 -> Divide1/2
  Constant24/1 -> Divide1/4
  Sqrt/1 -> Divide1/3
  Constant1/1 -> Sqrt/1
  Divide1/1 -> Divide/2
  Divide/1 -> MATLAB Function1/3(L_Iq), Divide2/1
  扭矩常量Kr  N/A/1 -> Divide2/2
  MATLAB Function/1(T) -> Gain1/1
  Data Store Read1/1 -> MATLAB Function1/2(Iq)
  Divide2/1 -> Gain/1
  Gain/1 -> Saturation1/1
  MATLAB Function1/1(T) -> Saturation2/1
  油压传感器/1 -> MATLAB Function/1(youya)
  Data Store Read3/1 -> MATLAB Function/4(wurenyouya)
  Data Store Read8/1 -> MATLAB Function/3(status)
  Data Store Read2/1 -> MATLAB Function/2(model)
  Data Store Read5/1 -> MATLAB Function/5(Negativ_T)
  Saturation/1 -> MATLAB Function1/1(er_T)
  Gain1/1 -> Saturation/1
  Saturation1/1 -> MATLAB Function1/4(L_er_T)
  Saturation2/1 -> T/1
  MATLAB Function2/1(y) -> Divide/1
  Data Store Read23/1 -> MATLAB Function2/4(model)
  Data Store Read4/1 -> MATLAB Function2/1(P)
  Data Store Read6/1 -> MATLAB Function2/2(P1)
  Data Store Read7/1 -> MATLAB Function2/3(P2)

== system finalcode/Subsystem/Tx/TX控制器/控制器发送/188右后1/算术平均值滤波 ArithmeticAverage5 ==
  In1 : Inport
  Constant : Constant  Value=10
  Divide : Product  Inputs=*/
  Sum of Elements : Sum  Inputs=+
  Tapped Delay : simulink/Discrete/Tapped Delay  vinit=0.0  samptime=-1  NumDelays=10  DelayOrder=Oldest  includeCurrent=off
  angle : Outport
  wires:
  Tapped Delay/1 -> Sum of Elements/1
  In1/1 -> Tapped Delay/1
  Divide/1 -> angle/1
  Sum of Elements/1 -> Divide/1
  Constant/1 -> Divide/2

== system finalcode/Subsystem/Tx/TX控制器/控制器发送/188右后1/能量回收功率限制 ==
  note: U
  note: Iq
  Constant1 : Constant  Value=2
  Constant24 : Constant  Value=1000
  Data Store Read1 : DataStoreRead  DataStoreName=er_T_rb
  Data Store Read2 : DataStoreRead  DataStoreName=match_model
  Data Store Read23 : DataStoreRead  DataStoreName=match_model
  Data Store Read25 : DataStoreRead  DataStoreName=er_v_rb
  Data Store Read3 : DataStoreRead  DataStoreName=oral_pressure_rightbehind
  Data Store Read4 : DataStoreRead  DataStoreName=Power_recovery
  Data Store Read5 : DataStoreRead  DataStoreName=Negativ_T
  Data Store Read6 : DataStoreRead  DataStoreName=Power_recovery_xunji
  Data Store Read7 : DataStoreRead  DataStoreName=Power_recovery_zhixian
  Data Store Read8 : DataStoreRead  DataStoreName=workstation_status
  Divide : Product  Inputs=*/
  Divide1 : Product  Inputs=***/
  Divide2 : Product  Inputs=**
  Gain : Gain  Gain=100
  MATLAB Function : MATLAB Function  TreatAsAtomicUnit=on
  MATLAB Function1 : MATLAB Function  TreatAsAtomicUnit=on
  MATLAB Function2 : MATLAB Function  TreatAsAtomicUnit=on
  Saturation : Saturate  UpperLimit=0  LowerLimit=-1200
  Saturation1 : Saturate  UpperLimit=1200  LowerLimit=-1200
  Saturation2 : Saturate  UpperLimit=0  LowerLimit=-1200
  Sqrt : Sqrt  SaturateOnIntegerOverflow=on
  扭矩常量Kr  N/A : Constant  Value=0.26
  油压传感器 : DataStoreRead  DataStoreName=ebszhidongyouya
  电压常数Ke V/kU/min : Constant  Value=18.8
  T : Outport
  wires:
  Data Store Read25/1 -> Divide1/1
  电压常数Ke V/kU/min/1 -> Divide1/2
  Constant24/1 -> Divide1/4
  Sqrt/1 -> Divide1/3
  Constant1/1 -> Sqrt/1
  Divide1/1 -> Divide/2
  Divide/1 -> MATLAB Function1/3(L_Iq), Divide2/1
  扭矩常量Kr  N/A/1 -> Divide2/2
  MATLAB Function/1(T) -> Saturation/1
  Data Store Read1/1 -> MATLAB Function1/2(Iq)
  Divide2/1 -> Gain/1
  Gain/1 -> Saturation1/1
  MATLAB Function1/1(T) -> Saturation2/1
  油压传感器/1 -> MATLAB Function/1(youya)
  Data Store Read3/1 -> MATLAB Function/4(wurenyouya)
  Data Store Read8/1 -> MATLAB Function/3(status)
  Data Store Read2/1 -> MATLAB Function/2(model)
  Data Store Read5/1 -> MATLAB Function/5(Negativ_T)
  Saturation/1 -> MATLAB Function1/1(er_T)
  Saturation1/1 -> MATLAB Function1/4(L_er_T)
  Saturation2/1 -> T/1
  Data Store Read4/1 -> MATLAB Function2/1(P)
  MATLAB Function2/1(y) -> Divide/1
  Data Store Read23/1 -> MATLAB Function2/4(model)
  Data Store Read6/1 -> MATLAB Function2/2(P1)
  Data Store Read7/1 -> MATLAB Function2/3(P2)

== system finalcode/Subsystem/Tx/TX控制器/控制器发送/189左后1/算术平均值滤波 ArithmeticAverage5 ==
  In1 : Inport
  Constant : Constant  Value=10
  Divide : Product  Inputs=*/
  Sum of Elements : Sum  Inputs=+
  Tapped Delay : simulink/Discrete/Tapped Delay  vinit=0.0  samptime=-1  NumDelays=10  DelayOrder=Oldest  includeCurrent=off
  angle : Outport
  wires:
  Tapped Delay/1 -> Sum of Elements/1
  In1/1 -> Tapped Delay/1
  Divide/1 -> angle/1
  Sum of Elements/1 -> Divide/1
  Constant/1 -> Divide/2

== system finalcode/Subsystem/Tx/TX控制器/控制器发送/189左后1/能量回收功率限制 ==
  note: U
  note: Iq
  Constant1 : Constant  Value=2
  Constant24 : Constant  Value=1000
  Data Store Read1 : DataStoreRead  DataStoreName=er_T_lb
  Data Store Read2 : DataStoreRead  DataStoreName=match_model
  Data Store Read23 : DataStoreRead  DataStoreName=match_model
  Data Store Read25 : DataStoreRead  DataStoreName=er_v_lb
  Data Store Read3 : DataStoreRead  DataStoreName=oral_pressure_leftbehind
  Data Store Read4 : DataStoreRead  DataStoreName=Power_recovery
  Data Store Read5 : DataStoreRead  DataStoreName=Negativ_T
  Data Store Read6 : DataStoreRead  DataStoreName=Power_recovery_xunji
  Data Store Read7 : DataStoreRead  DataStoreName=Power_recovery_zhixian
  Data Store Read8 : DataStoreRead  DataStoreName=workstation_status
  Divide : Product  Inputs=*/
  Divide1 : Product  Inputs=***/
  Divide2 : Product  Inputs=**
  Gain : Gain  Gain=100
  MATLAB Function : MATLAB Function  TreatAsAtomicUnit=on
  MATLAB Function1 : MATLAB Function  TreatAsAtomicUnit=on
  MATLAB Function2 : MATLAB Function  TreatAsAtomicUnit=on
  Saturation : Saturate  UpperLimit=0  LowerLimit=-1200
  Saturation1 : Saturate  UpperLimit=1200  LowerLimit=-1200
  Saturation2 : Saturate  UpperLimit=0  LowerLimit=-1200
  Sqrt : Sqrt  SaturateOnIntegerOverflow=on
  扭矩常量Kr  N/A : Constant  Value=0.26
  油压传感器 : DataStoreRead  DataStoreName=ebszhidongyouya
  电压常数Ke V/kU/min : Constant  Value=18.8
  T : Outport
  wires:
  Data Store Read25/1 -> Divide1/1
  电压常数Ke V/kU/min/1 -> Divide1/2
  Constant24/1 -> Divide1/4
  Sqrt/1 -> Divide1/3
  Constant1/1 -> Sqrt/1
  Divide1/1 -> Divide/2
  Divide/1 -> MATLAB Function1/3(L_Iq), Divide2/1
  扭矩常量Kr  N/A/1 -> Divide2/2
  MATLAB Function/1(T) -> Saturation/1
  Data Store Read1/1 -> MATLAB Function1/2(Iq)
  Divide2/1 -> Gain/1
  Gain/1 -> Saturation1/1
  MATLAB Function1/1(T) -> Saturation2/1
  油压传感器/1 -> MATLAB Function/1(youya)
  Data Store Read3/1 -> MATLAB Function/4(wurenyouya)
  Data Store Read8/1 -> MATLAB Function/3(status)
  Data Store Read2/1 -> MATLAB Function/2(model)
  Data Store Read5/1 -> MATLAB Function/5(Negativ_T)
  Saturation/1 -> MATLAB Function1/1(er_T)
  Saturation1/1 -> MATLAB Function1/4(L_er_T)
  Saturation2/1 -> T/1
  MATLAB Function2/1(y) -> Divide/1
  Data Store Read4/1 -> MATLAB Function2/1(P)
  Data Store Read6/1 -> MATLAB Function2/2(P1)
  Data Store Read23/1 -> MATLAB Function2/4(model)
  Data Store Read7/1 -> MATLAB Function2/3(P2)
